simulink model "Task_No6_Thermal"  (R2023b)
settings: Solver=ode5  StartTime=0.0  StopTime=3600*24*7  FixedStep=1  RelTol=1e-3
InitFcn:
  | PARAMETERS;
StartFcn:
  | PARAMETERS;
values from neighbouring files (symbols this model uses):
  Conv_C_to_K = 273.15    [PARAMETERS.m]
  P_AC_AIR_FLOW = 1    [PARAMETERS.m]
  P_AREA_BATH = 2*4    (= 8)    [PARAMETERS.m]
  P_AREA_BDR1 = 3.87^2    (= 14.9769)    [PARAMETERS.m]
  P_AREA_BDR2 = 3.87*4.5    (= 17.415)    [PARAMETERS.m]
  P_AREA_EAST_WALL_BATH = 2*P_RM_HEIGHT - P_AREA_WIN_BATH    (= 3.7)    [PARAMETERS.m]
  P_AREA_EAST_WALL_BDR2 = 3.87*P_RM_HEIGHT - P_AREA_WIN_BDRS    (= 7.075)    [PARAMETERS.m]
  P_AREA_EAST_WALL_KIT = 4.13*P_RM_HEIGHT    (= 10.325)    [PARAMETERS.m]
  P_AREA_HALL = 2*6    (= 12)    [PARAMETERS.m]
  P_AREA_KIT = 4.13*4    (= 16.52)    [PARAMETERS.m]
  P_AREA_LVR = 4.13*6    (= 24.78)    [PARAMETERS.m]
  P_AREA_NORTH_WALL_BATH = 1.63*P_RM_HEIGHT    (= 4.075)    [PARAMETERS.m]
  P_AREA_NORTH_WALL_BDR1 = 3.87*P_RM_HEIGHT - P_AREA_WIN_BDRS    (= 7.075)    [PARAMETERS.m]
  P_AREA_NORTH_WALL_BDR2 = 4.5*P_RM_HEIGHT - P_AREA_WIN_BDRS    (= 8.65)    [PARAMETERS.m]
  P_AREA_OUTER_WALL_BATH = (1.63+2)*P_RM_HEIGHT - P_AREA_WIN_BATH    (= 7.775)    [PARAMETERS.m]
  P_AREA_OUTER_WALL_BDR1 = 3.87*2*P_RM_HEIGHT - P_AREA_WIN_BDRS    (= 16.75)    [PARAMETERS.m]
  P_AREA_OUTER_WALL_BDR2 = (4.5+3.87)*P_RM_HEIGHT - P_AREA_WIN_BDRS*2    (= 15.725)    [PARAMETERS.m]
  P_AREA_OUTER_WALL_HALL = 2*P_RM_HEIGHT - P_AREA_SING_DOOR    (= 2.9)    [PARAMETERS.m]
  P_AREA_OUTER_WALL_KIT = (4+4.13)*P_RM_HEIGHT - P_AREA_WIN_KIT    (= 13.725)    [PARAMETERS.m]
  P_AREA_OUTER_WALL_LVR = (4.13+6)*P_RM_HEIGHT - P_AREA_WIN_LVR    (= 14.325)    [PARAMETERS.m]
  P_AREA_SOUTH_WALL_KIT = 4*P_RM_HEIGHT - P_AREA_WIN_KIT    (= 3.4)    [PARAMETERS.m]
  P_AREA_SOUTH_WALL_LVR = 6*P_RM_HEIGHT - P_AREA_WIN_LVR    (= 4)    [PARAMETERS.m]
  P_AREA_WALL_BATH_KIT = 4*P_RM_HEIGHT    (= 10)    [PARAMETERS.m]
  P_AREA_WALL_BDR1_BDR2 = 3.87*P_RM_HEIGHT    (= 9.675)    [PARAMETERS.m]
  P_AREA_WALL_BDR1_HALL = 3.87*P_RM_HEIGHT - P_AREA_SING_DOOR    (= 7.575)    [PARAMETERS.m]
  P_AREA_WALL_BDR2_BATH = 2.37*P_RM_HEIGHT    (= 5.925)    [PARAMETERS.m]
  P_AREA_WALL_BDR2_HALL = 2.13*P_RM_HEIGHT - P_AREA_SING_DOOR    (= 3.225)    [PARAMETERS.m]
  P_AREA_WALL_HALL_BATH = 2*P_RM_HEIGHT - P_AREA_SING_DOOR    (= 2.9)    [PARAMETERS.m]
  P_AREA_WALL_HALL_LVR = 6*P_RM_HEIGHT - P_AREA_DBL_DOOR    (= 10.8)    [PARAMETERS.m]
  P_AREA_WALL_LVR_KIT = 4.13*P_RM_HEIGHT - P_AREA_DBL_DOOR    (= 6.125)    [PARAMETERS.m]
  P_AREA_WIN_BATH = P_H_WIN_NORM*P_W_WIN_BATH    (= 1.3)    [PARAMETERS.m]
  P_AREA_WIN_BDRS = P_H_WIN_NORM*P_W_WIN_BDRS    (= 2.6)    [PARAMETERS.m]
  P_AREA_WIN_KIT = P_H_WIN_DOOR*P_W_WIN_KIT    (= 6.6)    [PARAMETERS.m]
  P_AREA_WIN_LVR = P_H_WIN_DOOR*P_W_WIN_LVR    (= 11)    [PARAMETERS.m]
  P_CP_AIR = 1012    [PARAMETERS.m]
  P_DENSITY_BRICK = 2/(10^-3)    (= 2000)    [PARAMETERS.m]
  P_DENSITY_PUR = 150    [PARAMETERS.m]
  P_EM_GLASS = 0.94    [PARAMETERS.m]
  P_EM_WALL = 0.94    [PARAMETERS.m]
  P_HUMAN = 60    [PARAMETERS.m]
  P_M_WINDOW_SPEC = 20    [PARAMETERS.m]
  P_THICK_BRICK = 0.175    [PARAMETERS.m]
  P_THICK_PUR = P_THICK_WALL - P_THICK_BRICK    (= 0.125)    [PARAMETERS.m]
  T_COOLER = 12    [PARAMETERS.m]
  T_HEATER = 50    [PARAMETERS.m]
  T_INIT_BDR = 22    [PARAMETERS.m]
  T_INIT_OUT = 2.9    [PARAMETERS.m]
  U_CEIL = 1.1    [PARAMETERS.m]
  U_INNER_WALL_BR = 3    [PARAMETERS.m]
  U_INNER_WALL_PC = 0.6    [PARAMETERS.m]
  U_WALL = 0.32    [PARAMETERS.m]
  U_WINDOW = 3.0    (= 3)    [PARAMETERS.m]
undefined symbols (not defined in the file or in its folder): TBL_SOL_EAST_01, TBL_SOL_EAST_02, TBL_SOL_EAST_03, TBL_SOL_EAST_04, TBL_SOL_EAST_05, TBL_SOL_EAST_06, TBL_SOL_EAST_07, TBL_SOL_EAST_08, TBL_SOL_EAST_09, TBL_SOL_EAST_10, TBL_SOL_EAST_11, TBL_SOL_EAST_12, TBL_SOL_NORTH_01, TBL_SOL_NORTH_02, TBL_SOL_NORTH_03, TBL_SOL_NORTH_04, TBL_SOL_NORTH_05, TBL_SOL_NORTH_06, TBL_SOL_NORTH_07, TBL_SOL_NORTH_08, TBL_SOL_NORTH_09, TBL_SOL_NORTH_10, TBL_SOL_NORTH_11, TBL_SOL_NORTH_12, TBL_SOL_SOUTH_01, TBL_TEMP
libraries: fl_lib x135, nesl_utility x39, slpidlib x3
(part 3 of 3)

== system Task_No6_Thermal/sub_House/Living Room/Heat source human ==
  Constant : Constant  Value=P_HUMAN
  Controlled Heat Flow Rate Source : fl_lib/Thermal/Thermal Sources/Controlled Heat Flow Rate Source
  Product : Product
  Simulink-PS Converter : nesl_utility/Simulink-PS Converter  PhysicalDomain=network_engine_domain  SubClassName=ps_input  LeftPortType=input  RightPortType=output  PseudoPeriodic=off  Frequencies=[]  NoiseDistribution=none  NoiseParameters=[]  Unit=1  AffineConversion=off  FilteringAndDerivatives=provide  SimscapeFilterOrder=1  InputFilterTimeConstant=0.001  UdotUserProvided=0
  Thermal Reference : fl_lib/Thermal/Thermal Elements/Thermal Reference
  Conn1 : PMIOPort  Side=Left
  wires:
  [N_LVR] -> Product/1
  Constant/1 -> Product/2
  Product/1 -> Simulink-PS Converter/1
  connections:
  Thermal Reference/LConn1 -- Controlled Heat Flow Rate Source/RConn2
  Simulink-PS Converter/RConn1 -- Controlled Heat Flow Rate Source/RConn1
  Controlled Heat Flow Rate Source/LConn1 -- Conn1/RConn1

== system Task_No6_Thermal/sub_House/Living Room/Inside Enivornment Temperature ==
  T_ENV : Inport
  Constant2 : Constant  Value=Conv_C_to_K
  Controlled Temperature Source : fl_lib/Thermal/Thermal Sources/Controlled Temperature Source
  Simulink-PS Converter1 : nesl_utility/Simulink-PS Converter  PhysicalDomain=network_engine_domain  SubClassName=ps_input  LeftPortType=input  RightPortType=output  PseudoPeriodic=off  Frequencies=[]  NoiseDistribution=none  NoiseParameters=[]  Unit=1  AffineConversion=off  FilteringAndDerivatives=provide  SimscapeFilterOrder=1  InputFilterTimeConstant=0.001  UdotUserProvided=0
  Sum : Sum  Inputs=|++
  Thermal Reference1 : fl_lib/Thermal/Thermal Elements/Thermal Reference
  Conn1 : PMIOPort  Side=Left
  wires:
  T_ENV/1 -> Sum/1
  Constant2/1 -> Sum/2
  Sum/1 -> Simulink-PS Converter1/1
  connections:
  Controlled Temperature Source/LConn1 -- Conn1/RConn1
  Simulink-PS Converter1/RConn1 -- Controlled Temperature Source/RConn1
  Thermal Reference1/LConn1 -- Controlled Temperature Source/RConn2

== system Task_No6_Thermal/sub_House/Living Room/Outside Temperature ==
  T_OUT : Inport
  Constant2 : Constant  Value=Conv_C_to_K
  Controlled Temperature Source : fl_lib/Thermal/Thermal Sources/Controlled Temperature Source
  Simulink-PS Converter1 : nesl_utility/Simulink-PS Converter  PhysicalDomain=network_engine_domain  SubClassName=ps_input  LeftPortType=input  RightPortType=output  PseudoPeriodic=off  Frequencies=[]  NoiseDistribution=none  NoiseParameters=[]  Unit=1  AffineConversion=off  FilteringAndDerivatives=provide  SimscapeFilterOrder=1  InputFilterTimeConstant=0.001  UdotUserProvided=0
  Sum : Sum  Inputs=|++
  Thermal Reference1 : fl_lib/Thermal/Thermal Elements/Thermal Reference
  Conn1 : PMIOPort  Side=Left
  wires:
  Sum/1 -> Simulink-PS Converter1/1
  Constant2/1 -> Sum/2
  T_OUT/1 -> Sum/1
  connections:
  Thermal Reference1/LConn1 -- Controlled Temperature Source/RConn2
  Simulink-PS Converter1/RConn1 -- Controlled Temperature Source/RConn1
  Controlled Temperature Source/LConn1 -- Conn1/RConn1

== system Task_No6_Thermal/sub_House/Living Room/SOLAR__WALL ==
  Constant : Constant  Value=P_AREA_SOUTH_WALL_LVR
  Constant1 : Constant  Value=P_EM_WALL
  Controlled Heat Flow Rate Source : fl_lib/Thermal/Thermal Sources/Controlled Heat Flow Rate Source
  Product : Product  Inputs=3
  Simulink-PS Converter : nesl_utility/Simulink-PS Converter  PhysicalDomain=network_engine_domain  SubClassName=ps_input  LeftPortType=input  RightPortType=output  PseudoPeriodic=off  Frequencies=[]  NoiseDistribution=none  NoiseParameters=[]  Unit=1  AffineConversion=off  FilteringAndDerivatives=provide  SimscapeFilterOrder=1  InputFilterTimeConstant=0.001  UdotUserProvided=0
  Thermal Reference : fl_lib/Thermal/Thermal Elements/Thermal Reference
  Conn1 : PMIOPort  Side=Left
  wires:
  Constant/1 -> Product/2
  Constant1/1 -> Product/1
  [SOL_SOUTH] -> Product/3
  Product/1 -> Simulink-PS Converter/1
  connections:
  Controlled Heat Flow Rate Source/LConn1 -- Conn1/RConn1
  Simulink-PS Converter/RConn1 -- Controlled Heat Flow Rate Source/RConn1
  Thermal Reference/LConn1 -- Controlled Heat Flow Rate Source/RConn2

== system Task_No6_Thermal/sub_House/Living Room/SOLAR__WINDOW ==
  Constant : Constant  Value=P_AREA_WIN_LVR
  Constant1 : Constant  Value=P_EM_GLASS
  Controlled Heat Flow Rate Source : fl_lib/Thermal/Thermal Sources/Controlled Heat Flow Rate Source
  Product : Product  Inputs=3
  Simulink-PS Converter : nesl_utility/Simulink-PS Converter  PhysicalDomain=network_engine_domain  SubClassName=ps_input  LeftPortType=input  RightPortType=output  PseudoPeriodic=off  Frequencies=[]  NoiseDistribution=none  NoiseParameters=[]  Unit=1  AffineConversion=off  FilteringAndDerivatives=provide  SimscapeFilterOrder=1  InputFilterTimeConstant=0.001  UdotUserProvided=0
  Thermal Reference : fl_lib/Thermal/Thermal Elements/Thermal Reference
  Conn1 : PMIOPort  Side=Left
  wires:
  Product/1 -> Simulink-PS Converter/1
  [SOL_SOUTH] -> Product/3
  Constant1/1 -> Product/1
  Constant/1 -> Product/2
  connections:
  Thermal Reference/LConn1 -- Controlled Heat Flow Rate Source/RConn2
  Simulink-PS Converter/RConn1 -- Controlled Heat Flow Rate Source/RConn1
  Controlled Heat Flow Rate Source/LConn1 -- Conn1/RConn1

== system Task_No6_Thermal/sub_House/Living Room/TEMP_01 ==
  Constant2 : Constant  Value=Conv_C_to_K
  PS-Simulink Converter : nesl_utility/PS-Simulink Converter  PhysicalDomain=network_engine_domain  SubClassName=ps_output  LeftPortType=input  RightPortType=output  PseudoPeriodic=off  Frequencies=[]  VectorFormat=inherit  Unit=inherit  AffineConversion=off
  Sum : Sum  Inputs=|+-
  Temperature Sensor : fl_lib/Thermal/Thermal Sensors/Temperature Sensor  temperature_measure=foundation.enum.MeasurementReference.difference
  Thermal Reference2 : fl_lib/Thermal/Thermal Elements/Thermal Reference
  PS : PMIOPort  Side=Left
  Sim : Outport
  wires:
  Constant2/1 -> Sum/2
  PS-Simulink Converter/1 -> Sum/1
  Sum/1 -> Sim/1
  connections:
  PS/RConn1 -- Temperature Sensor/LConn1
  PS-Simulink Converter/LConn1 -- Temperature Sensor/RConn2
  Thermal Reference2/LConn1 -- Temperature Sensor/RConn1

== system Task_No6_Thermal/sub_House/Living Room/Wall (LVR<->Outside) ==
  InAir-Wall : fl_lib/Thermal/Thermal Elements/Thermal Resistance  resistance=1/(U_WALL*P_AREA_OUTER_WALL_LVR)/2 K/W  T_specify=off  T_priority=None  T=0 K  T_nominal_specify=off  T_nominal_unit=K  T_nominal_value=1  Q_specify=off  Q_priority=None  Q=0 W  Q_nominal_specify=off  Q_nominal_unit=W  Q_nominal_value=1
  Thermal Mass of wall : fl_lib/Thermal/Thermal Elements/Thermal Mass  mass_type=foundation.enum.constant_variable.constant  mass=P_AREA_OUTER_WALL_LVR*(P_THICK_BRICK*P_DENSITY_BRICK+P_THICK_PUR*P_DENSITY_PUR) kg  sp_heat=P_CP_WALL J/(K*kg)  mass_min=1e-6 kg  num_ports=foundation.enum.numPorts2.one  m_specify=off  m_priority=High  m=1 kg  m_nominal_specify=off  m_nominal_unit=kg  m_nominal_value=1  T_specify=on  T_priority=High  T=T_INIT_BDR degC  T_nominal_specify=off  T_nominal_unit=K  T_nominal_value=1  Q_specify=off  Q_priority=None  Q=0 W  Q_nominal_specify=off  Q_nominal_unit=W  Q_nominal_value=1
  Wall-OutAir : fl_lib/Thermal/Thermal Elements/Thermal Resistance  resistance=1/(U_WALL*P_AREA_OUTER_WALL_LVR)/2 K/W  T_specify=off  T_priority=None  T=0 K  T_nominal_specify=off  T_nominal_unit=K  T_nominal_value=1  Q_specify=off  Q_priority=None  Q=0 W  Q_nominal_specify=off  Q_nominal_unit=W  Q_nominal_value=1
  Conn1 : PMIOPort  Side=Left
  Conn3 : PMIOPort  Port=2  Side=Right
  Conn2 : PMIOPort  Port=3  Side=Right
  connections:
  Wall-OutAir/RConn1 -- Conn2/RConn1
  Wall-OutAir/LConn1 -- Conn3/RConn1 -- Thermal Mass of wall/LConn1 -- InAir-Wall/RConn1
  Conn1/RConn1 -- InAir-Wall/LConn1

== system Task_No6_Thermal/sub_House/Living Room/Window (LVR<->Outside) ==
  InAir-Window : fl_lib/Thermal/Thermal Elements/Thermal Resistance  resistance=1/(U_WINDOW*P_AREA_WIN_LVR)/2 K/W  T_specify=off  T_priority=None  T=0 K  T_nominal_specify=off  T_nominal_unit=K  T_nominal_value=1  Q_specify=off  Q_priority=None  Q=0 W  Q_nominal_specify=off  Q_nominal_unit=W  Q_nominal_value=1
  Thermal Mass of window : fl_lib/Thermal/Thermal Elements/Thermal Mass  mass_type=foundation.enum.constant_variable.constant  mass=P_M_WINDOW_SPEC*P_AREA_WIN_LVR kg  sp_heat=P_CP_GLASS J/(K*kg)  mass_min=1e-6 kg  num_ports=foundation.enum.numPorts2.one  m_specify=off  m_priority=High  m=1 kg  m_nominal_specify=off  m_nominal_unit=kg  m_nominal_value=1  T_specify=on  T_priority=High  T=T_INIT_BDR degC  T_nominal_specify=off  T_nominal_unit=K  T_nominal_value=1  Q_specify=off  Q_priority=None  Q=0 W  Q_nominal_specify=off  Q_nominal_unit=W  Q_nominal_value=1
  Window-OutAir : fl_lib/Thermal/Thermal Elements/Thermal Resistance  resistance=1/(U_WINDOW*P_AREA_WIN_LVR)/2 K/W  T_specify=off  T_priority=None  T=0 K  T_nominal_specify=off  T_nominal_unit=K  T_nominal_value=1  Q_specify=off  Q_priority=None  Q=0 W  Q_nominal_specify=off  Q_nominal_unit=W  Q_nominal_value=1
  Conn1 : PMIOPort  Side=Right
  Conn2 : PMIOPort  Port=2  Side=Left
  Conn3 : PMIOPort  Port=3  Side=Right
  connections:
  Conn2/RConn1 -- InAir-Window/LConn1
  Conn1/RConn1 -- Window-OutAir/RConn1
  InAir-Window/RConn1 -- Conn3/RConn1 -- Thermal Mass of window/LConn1 -- Window-OutAir/LConn1

== system Task_No6_Thermal/sub_House/Bedroom 1/AirConditioning/AC_scheduling ==
  In1 : Inport
  In3 : Inport  Port=2
  In2 : Inport  Port=3
  Constant : Constant  Value=0
  Constant1 : Constant  Value=0
  Constant2 : Constant
  Product : Product
  Switch : Switch  Criteria=u2 > Threshold  SaturateOnIntegerOverflow=off  InputSameDT=off
  Switch1 : Switch  Criteria=u2 > Threshold  SaturateOnIntegerOverflow=off  InputSameDT=off
  Switch2 : Switch  Criteria=u2 > Threshold  SaturateOnIntegerOverflow=off  InputSameDT=off
  Out1 : Outport
  wires:
  Product/1 -> Switch1/3
  Constant1/1 -> Switch/3
  In2/1 -> Switch1/1, Product/1
  [N_BDR1] -> Switch/2
  Switch/1 -> Product/2
  Constant2/1 -> Switch/1
  Constant/1 -> Switch2/3
  In1/1 -> Switch2/2
  Switch2/1 -> Out1/1
  Switch1/1 -> Switch2/1
  In3/1 -> Switch1/2

== system Task_No6_Thermal/sub_House/Bedroom 1/AirConditioning/sub_AC ==
  SWITCH : Inport
  AC Unit (PI) : slpidlib/PID Controller  Controller=PI  Form=Parallel  TimeDomain=Continuous-time  UseExternalTs=off  SampleTime=-1  IntegratorMethod=Forward Euler  FilterMethod=Forward Euler  ControllerParametersSource=internal  P=0.273405653956394  I=0.00661922856888281  UseKiTs=off  D=39.5738922859411  N=3204.37920267902  UseFilter=on  TunerSelectOption=Transfer Function Based (PID Tuner App)  InitialConditionSource=internal  InitialConditionForIntegrator=0  InitialConditionForFilter=0  DifferentiatorICPrevScaledInput=0  ExternalReset=none  TrackingMode=off  Kt=1  LimitOutput=on  SatLimitsSource=internal  UpperSaturationLimit=1  LowerSaturationLimit=-1  LinearizeAsGain=on  AntiWindupMode=clamping  Kb=1  LimitIntegrator=off  UpperIntegratorSaturationLimit=inf  LowerIntegratorSaturationLimit=-inf  POutMin=[]  POutMax=[]  IOutMin=[]  IOutMax=[]  DOutMin=[]  DOutMax=[]  NOutMin=[]  NOutMax=[]  SumOutMin=[]  SumOutMax=[]  SaturationOutMin=[]  SaturationOutMax=[]  PParamMin=[]  PParamMax=[]  IParamMin=[]  IParamMax=[]  DParamMin=[]  DParamMax=[]  NParamMin=[]  NParamMax=[]  KbParamMin=[]  KbParamMax=[]  KtParamMin=[]  KtParamMax=[]  KbOutMin=[]  KbOutMax=[]  KtOutMin=[]  KtOutMax=[]  IntegratorOutMin=[]  IntegratorOutMax=[]  FilterOutMin=[]  FilterOutMax=[]  SumI1OutMin=[]  SumI1OutMax=[]  SumI2OutMin=[]  SumI2OutMax=[]  SumI3OutMin=[]  SumI3OutMax=[]  SumI4OutMin=[]  SumI4OutMax=[]  SumDOutMin=[]  SumDOutMax=[]  DifferentiatorOutMin=[]  DifferentiatorOutMax=[]  FilterDiffOutCoefMin=[]  FilterDiffOutCoefMax=[]  ReciprocalOutMin=[]  ReciprocalOutMax=[]  SumDenOutMin=[]  SumDenOutMax=[]  SumNumOutMin=[]  SumNumOutMax=[]  DivideOutMin=[]  DivideOutMax=[]  UdiffTsProdOutMin=[]  UdiffTsProdOutMax=[]  NTsProdOutMin=[]  NTsProdOutMax=[]  UintegralTsProdOutMin=[]  UintegralTsProdOutMax=[]  UngainTsProdOutMin=[]  UngainTsProdOutMax=[]  ClampingZeroOutDataTypeStr=Inherit: Inherit via back propagation  ClampingZeroOutMin=[]  ClampingZeroOutMax=[]  FilterDenConstantOutDataTypeStr=Inherit: Inherit via back propagation  FilterDenConstantOutMin=[]  FilterDenConstantOutMax=[]  PCopyOutDataTypeStr=Inherit: Inherit via back propagation  PCopyOutMin=[]  PCopyOutMax=[]  NCopyOutDataTypeStr=Inherit: Inherit via back propagation  NCopyOutMin=[]  NCopyOutMax=[]  IntegratorContinuousStateAttributes=''  IntegratorStateMustResolveToSignalObject=off  IntegratorRTWStateStorageClass=Auto  FilterContinuousStateAttributes=''  FilterStateMustResolveToSignalObject=off  FilterRTWStateStorageClass=Auto  ParallelPVariant=InternalParameters  IdealPVariant=Disabled  IVariant=InternalParameters  DVariant=Disabled  IntegratorVariant=Continuous  SatVariant=Enabled  AWVariant=ContClampingParallel  PCopyVariant=Disabled  TRVariant=Disabled  FdbkBlocksVariant=Forward  IdealPFdbkVariant=Disabled  SatFdbkVariant=Disabled  DerivativeFilterVariant=Disabled  NVariant=Disabled  NCopyVariant=Disabled_SignalSpec  FilterICVariant=Disabled  IntegratorICVariant=InternalICs  ExternalResetVariant=Disabled  TRSumVariant=Passthrough  SumFdbkVariant=Disabled  SumVariant=Sum_PI  TsampFilterVariant=InternalTs  TsampNgainVariant=Passthrough  TsampIntegralVariant=Disabled_SignalSpec  ExternalSaturationOutDataTypeStr=Inherit: Same as second input
  Gain : Gain  Gain=-1
  Saturation : Saturate  UpperLimit=1  LowerLimit=0
  Saturation1 : Saturate  UpperLimit=1  LowerLimit=0
  HEAT : Outport
  COOLING : Outport  Port=2
  wires:
  Gain/1 -> Saturation1/1
  Saturation1/1 -> COOLING/1
  AC Unit (PI)/1 -> Gain/1, Saturation/1  "SWITCH"
  Saturation/1 -> HEAT/1
  SWITCH/1 -> AC Unit (PI)/1

== system Task_No6_Thermal/sub_House/Bedroom 1/AirConditioning/sub_Cooling ==
  SWITCH : Inport
  T_BDR : Inport  Port=2
  Constant2 : Constant  Value=T_COOLER
  Gain : Gain  Gain=P_CP_AIR*P_AC_AIR_FLOW
  Product : Product
  Sum : Sum  Inputs=|-+
  Transfer Fcn : TransferFcn  Denominator=[1 1]
  P_COOL : Outport
  wires:
  Product/1 -> Transfer Fcn/1  "P_HEAT"
  T_BDR/1 -> Sum/1
  Gain/1 -> Product/2  "P_HEAT"
  SWITCH/1 -> Product/1
  Constant2/1 -> Sum/2  "T_HEATER"
  Transfer Fcn/1 -> P_COOL/1  "P_HEAT"
  Sum/1 -> Gain/1  "DELTA_T"

== system Task_No6_Thermal/sub_House/Bedroom 1/AirConditioning/sub_Heating ==
  SWITCH : Inport
  T_BDR : Inport  Port=2
  Constant2 : Constant  Value=T_HEATER
  Gain : Gain  Gain=P_CP_AIR*P_AC_AIR_FLOW
  Product : Product
  Sum : Sum  Inputs=|-+
  Transfer Fcn : TransferFcn  Denominator=[1 1]
  P_HEAT : Outport
  wires:
  Sum/1 -> Gain/1  "DELTA_T"
  Transfer Fcn/1 -> P_HEAT/1  "P_HEAT"
  Constant2/1 -> Sum/2  "T_HEATER"
  SWITCH/1 -> Product/1
  Gain/1 -> Product/2  "P_HEAT"
  T_BDR/1 -> Sum/1
  Product/1 -> Transfer Fcn/1  "P_HEAT"

== system Task_No6_Thermal/sub_House/Bedroom 2/AirConditioning/AC_scheduling1 ==
  In1 : Inport
  In3 : Inport  Port=2
  In2 : Inport  Port=3
  Constant : Constant  Value=0
  Constant1 : Constant  Value=0
  Constant2 : Constant
  Product : Product
  Switch : Switch  Criteria=u2 > Threshold  SaturateOnIntegerOverflow=off  InputSameDT=off
  Switch1 : Switch  Criteria=u2 > Threshold  SaturateOnIntegerOverflow=off  InputSameDT=off
  Switch2 : Switch  Criteria=u2 > Threshold  SaturateOnIntegerOverflow=off  InputSameDT=off
  SWITCH : Outport
  wires:
  Product/1 -> Switch1/3
  Constant1/1 -> Switch/3
  In2/1 -> Switch1/1, Product/1
  [N_BDR1] -> Switch/2
  Switch/1 -> Product/2
  Constant2/1 -> Switch/1
  Constant/1 -> Switch2/3
  In1/1 -> Switch2/2
  Switch2/1 -> SWITCH/1
  Switch1/1 -> Switch2/1
  In3/1 -> Switch1/2

== system Task_No6_Thermal/sub_House/Bedroom 2/AirConditioning/sub_AC ==
  SWITCH : Inport
  AC Unit (PI) : slpidlib/PID Controller  Controller=PI  Form=Parallel  TimeDomain=Continuous-time  UseExternalTs=off  SampleTime=-1  IntegratorMethod=Forward Euler  FilterMethod=Forward Euler  ControllerParametersSource=internal  P=0.273405653956394  I=0.00661922856888281  UseKiTs=off  D=39.5738922859411  N=3204.37920267902  UseFilter=on  TunerSelectOption=Transfer Function Based (PID Tuner App)  InitialConditionSource=internal  InitialConditionForIntegrator=0  InitialConditionForFilter=0  DifferentiatorICPrevScaledInput=0  ExternalReset=none  TrackingMode=off  Kt=1  LimitOutput=on  SatLimitsSource=internal  UpperSaturationLimit=1  LowerSaturationLimit=-1  LinearizeAsGain=on  AntiWindupMode=clamping  Kb=1  LimitIntegrator=off  UpperIntegratorSaturationLimit=inf  LowerIntegratorSaturationLimit=-inf  POutMin=[]  POutMax=[]  IOutMin=[]  IOutMax=[]  DOutMin=[]  DOutMax=[]  NOutMin=[]  NOutMax=[]  SumOutMin=[]  SumOutMax=[]  SaturationOutMin=[]  SaturationOutMax=[]  PParamMin=[]  PParamMax=[]  IParamMin=[]  IParamMax=[]  DParamMin=[]  DParamMax=[]  NParamMin=[]  NParamMax=[]  KbParamMin=[]  KbParamMax=[]  KtParamMin=[]  KtParamMax=[]  KbOutMin=[]  KbOutMax=[]  KtOutMin=[]  KtOutMax=[]  IntegratorOutMin=[]  IntegratorOutMax=[]  FilterOutMin=[]  FilterOutMax=[]  SumI1OutMin=[]  SumI1OutMax=[]  SumI2OutMin=[]  SumI2OutMax=[]  SumI3OutMin=[]  SumI3OutMax=[]  SumI4OutMin=[]  SumI4OutMax=[]  SumDOutMin=[]  SumDOutMax=[]  DifferentiatorOutMin=[]  DifferentiatorOutMax=[]  FilterDiffOutCoefMin=[]  FilterDiffOutCoefMax=[]  ReciprocalOutMin=[]  ReciprocalOutMax=[]  SumDenOutMin=[]  SumDenOutMax=[]  SumNumOutMin=[]  SumNumOutMax=[]  DivideOutMin=[]  DivideOutMax=[]  UdiffTsProdOutMin=[]  UdiffTsProdOutMax=[]  NTsProdOutMin=[]  NTsProdOutMax=[]  UintegralTsProdOutMin=[]  UintegralTsProdOutMax=[]  UngainTsProdOutMin=[]  UngainTsProdOutMax=[]  ClampingZeroOutDataTypeStr=Inherit: Inherit via back propagation  ClampingZeroOutMin=[]  ClampingZeroOutMax=[]  FilterDenConstantOutDataTypeStr=Inherit: Inherit via back propagation  FilterDenConstantOutMin=[]  FilterDenConstantOutMax=[]  PCopyOutDataTypeStr=Inherit: Inherit via back propagation  PCopyOutMin=[]  PCopyOutMax=[]  NCopyOutDataTypeStr=Inherit: Inherit via back propagation  NCopyOutMin=[]  NCopyOutMax=[]  IntegratorContinuousStateAttributes=''  IntegratorStateMustResolveToSignalObject=off  IntegratorRTWStateStorageClass=Auto  FilterContinuousStateAttributes=''  FilterStateMustResolveToSignalObject=off  FilterRTWStateStorageClass=Auto  ParallelPVariant=InternalParameters  IdealPVariant=Disabled  IVariant=InternalParameters  DVariant=Disabled  IntegratorVariant=Continuous  SatVariant=Enabled  AWVariant=ContClampingParallel  PCopyVariant=Disabled  TRVariant=Disabled  FdbkBlocksVariant=Forward  IdealPFdbkVariant=Disabled  SatFdbkVariant=Disabled  DerivativeFilterVariant=Disabled  NVariant=Disabled  NCopyVariant=Disabled_SignalSpec  FilterICVariant=Disabled  IntegratorICVariant=InternalICs  ExternalResetVariant=Disabled  TRSumVariant=Passthrough  SumFdbkVariant=Disabled  SumVariant=Sum_PI  TsampFilterVariant=InternalTs  TsampNgainVariant=Passthrough  TsampIntegralVariant=Disabled_SignalSpec  ExternalSaturationOutDataTypeStr=Inherit: Same as second input
  Gain : Gain  Gain=-1
  Saturation : Saturate  UpperLimit=1  LowerLimit=0
  Saturation1 : Saturate  UpperLimit=1  LowerLimit=0
  HEAT : Outport
  COOLING : Outport  Port=2
  wires:
  Gain/1 -> Saturation1/1
  Saturation1/1 -> COOLING/1
  AC Unit (PI)/1 -> Gain/1, Saturation/1  "SWITCH"
  Saturation/1 -> HEAT/1
  SWITCH/1 -> AC Unit (PI)/1

== system Task_No6_Thermal/sub_House/Bedroom 2/AirConditioning/sub_Cooling ==
  SWITCH : Inport
  T_BDR : Inport  Port=2
  Constant2 : Constant  Value=T_COOLER
  Gain : Gain  Gain=P_CP_AIR*P_AC_AIR_FLOW
  Product : Product
  Sum : Sum  Inputs=|-+
  Transfer Fcn : TransferFcn  Denominator=[1 1]
  P_COOL : Outport
  wires:
  Product/1 -> Transfer Fcn/1  "P_HEAT"
  T_BDR/1 -> Sum/1
  Gain/1 -> Product/2  "P_HEAT"
  SWITCH/1 -> Product/1
  Constant2/1 -> Sum/2  "T_HEATER"
  Transfer Fcn/1 -> P_COOL/1  "P_HEAT"
  Sum/1 -> Gain/1  "DELTA_T"

== system Task_No6_Thermal/sub_House/Bedroom 2/AirConditioning/sub_Heating ==
  SWITCH : Inport
  T_BDR : Inport  Port=2
  Constant2 : Constant  Value=T_HEATER
  Gain : Gain  Gain=P_CP_AIR*P_AC_AIR_FLOW
  Product : Product
  Sum : Sum  Inputs=|-+
  Transfer Fcn : TransferFcn  Denominator=[1 1]
  P_HEAT : Outport
  wires:
  Sum/1 -> Gain/1  "DELTA_T"
  Transfer Fcn/1 -> P_HEAT/1  "P_HEAT"
  Constant2/1 -> Sum/2  "T_HEATER"
  SWITCH/1 -> Product/1
  Gain/1 -> Product/2  "P_HEAT"
  T_BDR/1 -> Sum/1
  Product/1 -> Transfer Fcn/1  "P_HEAT"

== system Task_No6_Thermal/sub_House/Living Room/AirConditioning/AC_scheduling1 ==
  In1 : Inport
  In3 : Inport  Port=2
  In2 : Inport  Port=3
  Constant : Constant  Value=0
  Constant1 : Constant  Value=0
  Constant2 : Constant
  Product : Product
  Switch : Switch  Criteria=u2 > Threshold  SaturateOnIntegerOverflow=off  InputSameDT=off
  Switch1 : Switch  Criteria=u2 > Threshold  SaturateOnIntegerOverflow=off  InputSameDT=off
  Switch2 : Switch  Criteria=u2 > Threshold  SaturateOnIntegerOverflow=off  InputSameDT=off
  SWITCH : Outport
  wires:
  Product/1 -> Switch1/3
  Constant1/1 -> Switch/3
  In2/1 -> Switch1/1, Product/1
  [N_BDR1] -> Switch/2
  Switch/1 -> Product/2
  Constant2/1 -> Switch/1
  Constant/1 -> Switch2/3
  In1/1 -> Switch2/2
  Switch2/1 -> SWITCH/1
  Switch1/1 -> Switch2/1
  In3/1 -> Switch1/2

== system Task_No6_Thermal/sub_House/Living Room/AirConditioning/sub_AC ==
  SWITCH : Inport
  AC Unit (PI) : slpidlib/PID Controller  Controller=PI  Form=Parallel  TimeDomain=Continuous-time  UseExternalTs=off  SampleTime=-1  IntegratorMethod=Forward Euler  FilterMethod=Forward Euler  ControllerParametersSource=internal  P=0.273405653956394  I=0.00661922856888281  UseKiTs=off  D=39.5738922859411  N=3204.37920267902  UseFilter=on  TunerSelectOption=Transfer Function Based (PID Tuner App)  InitialConditionSource=internal  InitialConditionForIntegrator=0  InitialConditionForFilter=0  DifferentiatorICPrevScaledInput=0  ExternalReset=none  TrackingMode=off  Kt=1  LimitOutput=on  SatLimitsSource=internal  UpperSaturationLimit=1  LowerSaturationLimit=-1  LinearizeAsGain=on  AntiWindupMode=clamping  Kb=1  LimitIntegrator=off  UpperIntegratorSaturationLimit=inf  LowerIntegratorSaturationLimit=-inf  POutMin=[]  POutMax=[]  IOutMin=[]  IOutMax=[]  DOutMin=[]  DOutMax=[]  NOutMin=[]  NOutMax=[]  SumOutMin=[]  SumOutMax=[]  SaturationOutMin=[]  SaturationOutMax=[]  PParamMin=[]  PParamMax=[]  IParamMin=[]  IParamMax=[]  DParamMin=[]  DParamMax=[]  NParamMin=[]  NParamMax=[]  KbParamMin=[]  KbParamMax=[]  KtParamMin=[]  KtParamMax=[]  KbOutMin=[]  KbOutMax=[]  KtOutMin=[]  KtOutMax=[]  IntegratorOutMin=[]  IntegratorOutMax=[]  FilterOutMin=[]  FilterOutMax=[]  SumI1OutMin=[]  SumI1OutMax=[]  SumI2OutMin=[]  SumI2OutMax=[]  SumI3OutMin=[]  SumI3OutMax=[]  SumI4OutMin=[]  SumI4OutMax=[]  SumDOutMin=[]  SumDOutMax=[]  DifferentiatorOutMin=[]  DifferentiatorOutMax=[]  FilterDiffOutCoefMin=[]  FilterDiffOutCoefMax=[]  ReciprocalOutMin=[]  ReciprocalOutMax=[]  SumDenOutMin=[]  SumDenOutMax=[]  SumNumOutMin=[]  SumNumOutMax=[]  DivideOutMin=[]  DivideOutMax=[]  UdiffTsProdOutMin=[]  UdiffTsProdOutMax=[]  NTsProdOutMin=[]  NTsProdOutMax=[]  UintegralTsProdOutMin=[]  UintegralTsProdOutMax=[]  UngainTsProdOutMin=[]  UngainTsProdOutMax=[]  ClampingZeroOutDataTypeStr=Inherit: Inherit via back propagation  ClampingZeroOutMin=[]  ClampingZeroOutMax=[]  FilterDenConstantOutDataTypeStr=Inherit: Inherit via back propagation  FilterDenConstantOutMin=[]  FilterDenConstantOutMax=[]  PCopyOutDataTypeStr=Inherit: Inherit via back propagation  PCopyOutMin=[]  PCopyOutMax=[]  NCopyOutDataTypeStr=Inherit: Inherit via back propagation  NCopyOutMin=[]  NCopyOutMax=[]  IntegratorContinuousStateAttributes=''  IntegratorStateMustResolveToSignalObject=off  IntegratorRTWStateStorageClass=Auto  FilterContinuousStateAttributes=''  FilterStateMustResolveToSignalObject=off  FilterRTWStateStorageClass=Auto  ParallelPVariant=InternalParameters  IdealPVariant=Disabled  IVariant=InternalParameters  DVariant=Disabled  IntegratorVariant=Continuous  SatVariant=Enabled  AWVariant=ContClampingParallel  PCopyVariant=Disabled  TRVariant=Disabled  FdbkBlocksVariant=Forward  IdealPFdbkVariant=Disabled  SatFdbkVariant=Disabled  DerivativeFilterVariant=Disabled  NVariant=Disabled  NCopyVariant=Disabled_SignalSpec  FilterICVariant=Disabled  IntegratorICVariant=InternalICs  ExternalResetVariant=Disabled  TRSumVariant=Passthrough  SumFdbkVariant=Disabled  SumVariant=Sum_PI  TsampFilterVariant=InternalTs  TsampNgainVariant=Passthrough  TsampIntegralVariant=Disabled_SignalSpec  ExternalSaturationOutDataTypeStr=Inherit: Same as second input
  Gain : Gain  Gain=-1
  Saturation : Saturate  UpperLimit=1  LowerLimit=0
  Saturation1 : Saturate  UpperLimit=1  LowerLimit=0
  HEAT : Outport
  COOLING : Outport  Port=2
  wires:
  Gain/1 -> Saturation1/1
  Saturation1/1 -> COOLING/1
  AC Unit (PI)/1 -> Gain/1, Saturation/1  "SWITCH"
  Saturation/1 -> HEAT/1
  SWITCH/1 -> AC Unit (PI)/1

== system Task_No6_Thermal/sub_House/Living Room/AirConditioning/sub_Cooling ==
  SWITCH : Inport
  T_BDR : Inport  Port=2
  Constant2 : Constant  Value=T_COOLER
  Gain : Gain  Gain=P_CP_AIR*P_AC_AIR_FLOW
  Product : Product
  Sum : Sum  Inputs=|-+
  Transfer Fcn : TransferFcn  Denominator=[1 1]
  P_COOL : Outport
  wires:
  Product/1 -> Transfer Fcn/1  "P_HEAT"
  T_BDR/1 -> Sum/1
  Gain/1 -> Product/2  "P_HEAT"
  SWITCH/1 -> Product/1
  Constant2/1 -> Sum/2  "T_HEATER"
  Transfer Fcn/1 -> P_COOL/1  "P_HEAT"
  Sum/1 -> Gain/1  "DELTA_T"

== system Task_No6_Thermal/sub_House/Living Room/AirConditioning/sub_Heating ==
  SWITCH : Inport
  T_BDR : Inport  Port=2
  Constant2 : Constant  Value=T_HEATER
  Gain : Gain  Gain=P_CP_AIR*P_AC_AIR_FLOW
  Product : Product
  Sum : Sum  Inputs=|-+
  Transfer Fcn : TransferFcn  Denominator=[1 1]
  P_HEAT : Outport
  wires:
  Sum/1 -> Gain/1  "DELTA_T"
  Transfer Fcn/1 -> P_HEAT/1  "P_HEAT"
  Constant2/1 -> Sum/2  "T_HEATER"
  SWITCH/1 -> Product/1
  Gain/1 -> Product/2  "P_HEAT"
  T_BDR/1 -> Sum/1
  Product/1 -> Transfer Fcn/1  "P_HEAT"

== matlab function Task_No6_Thermal/sub_TOUT/Hour Loop Counter ==
  data: h input; h output
function h = Counter(h)

if h < 24
    h = h + 1/3600;
else
    h = 0;
end

== matlab function Task_No6_Thermal/sub_DailyRoutine/Time of day ==
  data: h input; h output; n_bdr1 output; n_bdr2 output; n_lvr output; n_kit output
function [h, n_bdr1, n_bdr2, n_lvr, n_kit] = day(h)

if h < 24*3600
    
    if h < 7*3600
        n_bdr1 = 2;
        n_bdr2 = 2;
        n_lvr = 0;
        n_kit = 0;
        h = h + 1;
    elseif h >= 7*3600 && h < 17*3600
        n_bdr1 = 0;
        n_bdr2 = 0;
        n_lvr = 1;
        n_kit = 0;
        h = h + 1;
    elseif h >= 17*3600 && h < 19*3600
        n_bdr1 = 2;
        n_bdr2 = 0;
        n_lvr = 0;
        n_kit = 2;
        h = h + 1;
    elseif h >= 19*3600 && h < 22*3600
        n_bdr1 = 0;
        n_bdr2 = 0;
        n_lvr = 4;
        n_kit = 0;
        h = h + 1;
    elseif h >= 22*3600 && h < 24*3600
        n_bdr1 = 2;
        n_bdr2 = 0;
        n_lvr = 2;
        n_kit = 0;
        h = h + 1;
    else
        n_bdr1 = 0;
        n_bdr2 = 0;
        n_lvr = 0;
        n_kit = 0;
        h = h + 1;
    end
else
    h = 0;
    n_bdr1 = 0;
    n_bdr2 = 0;
    n_lvr = 0;
    n_kit = 0;
end
